simulink model "switching_simulink"  (R2018a)
settings: Solver=VariableStepAuto  StartTime=0.0  StopTime=0.04  RelTol=1e-3
undefined symbols (not defined in the file or in its folder): carrier_phase, ffund, fundemental_phase, load_phase, ModulationIndex, Phase_Current, sampleTime
libraries: simulink x1, powerlib_meascontrol x1
settings Model: Creator=enes_  LastModifiedBy=enes_

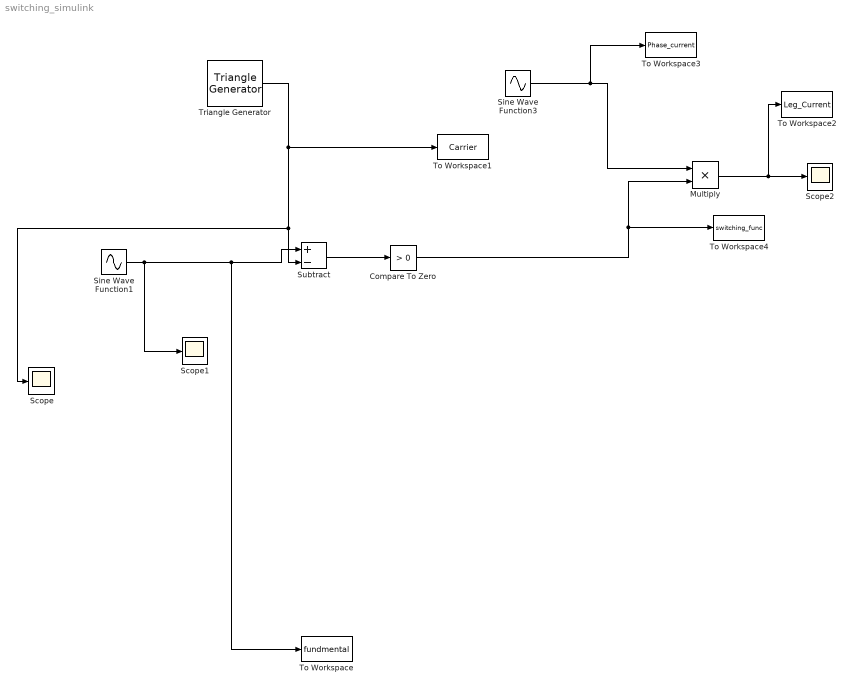
== system switching_simulink ==
  Compare To Zero : simulink/Logic and Bit Operations/Compare To Zero  relop=>  OutDataTypeStr=uint8
  Multiply : Product
  Scope : Scope
  Scope1 : Scope
  Scope2 : Scope
  Sine Wave Function1 : Sin  Amplitude=ModulationIndex  Frequency=ffund*2*pi  Phase=fundemental_phase  SampleTime=0
  Sine Wave Function3 : Sin  Amplitude=Phase_Current  Frequency=ffund*2*pi  Phase=load_phase+fundemental_phase  SampleTime=0
  Subtract : Sum  Inputs=+-
  To Workspace : ToWorkspace  VariableName=fundmental  SaveFormat=Timeseries  SampleTime=-1
  To Workspace1 : ToWorkspace  VariableName=Carrier  SaveFormat=Timeseries  SampleTime=-1
  To Workspace2 : ToWorkspace  VariableName=Leg_Current  SaveFormat=Timeseries  SampleTime=-1
  To Workspace3 : ToWorkspace  VariableName=Phase_current  SaveFormat=Timeseries  SampleTime=-1
  To Workspace4 : ToWorkspace  VariableName=switching_func  SaveFormat=Timeseries  SampleTime=-1
  Triangle Generator : powerlib_meascontrol/Pulse & Signal Generators/Triangle Generator  Freq=fsw  Phase=carrier_phase*180/pi  Ts=sampleTime
  wires:
  Compare To Zero/1 -> To Workspace4/1, Multiply/2
  Triangle Generator/1 -> To Workspace1/1, Scope/1, Subtract/2
  Subtract/1 -> Compare To Zero/1
  Sine Wave Function1/1 -> To Workspace/1, Subtract/1, Scope1/1
  Sine Wave Function3/1 -> To Workspace3/1, Multiply/1
  Multiply/1 -> To Workspace2/1, Scope2/1
